simulink model "RC"  (R2020a)
settings: Solver=VariableStepAuto  StartTime=0.0  StopTime=30  FixedStep=0.2  RelTol=1e-3
values from neighbouring files (symbols this model uses):
  a = a+1    (= 1)    [rc_model.m]
  c = 1/10*10^-6    (= 1e-07)    [rc_model.m]
  r = 10    [rc_model.m]
settings Model: Creator=I3  LastModifiedBy=I3

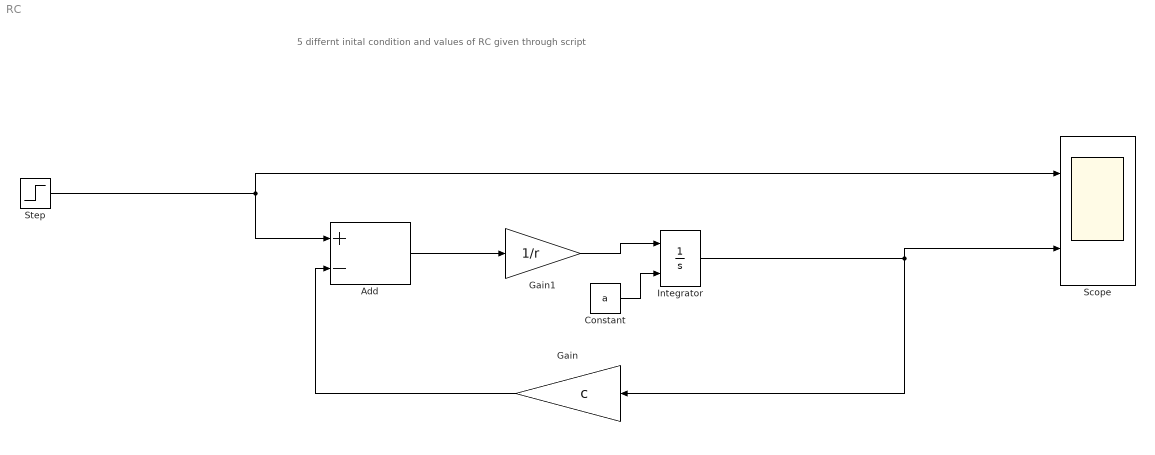
== system RC ==
  note: 5 differnt inital condition and values of RC given through script
  Add : Sum  Inputs=+-
  Constant : Constant  Value=a
  Gain : Gain  Gain=c
  Gain1 : Gain  Gain=1/r
  Integrator : Integrator  InitialConditionSource=external
  Scope : Scope  NumInputPorts=2
  Step : Step  SampleTime=0
  wires:
  Add/1 -> Gain1/1
  Integrator/1 -> Gain/1, Scope/2
  Gain/1 -> Add/2
  Gain1/1 -> Integrator/1
  Step/1 -> Scope/1, Add/1
  Constant/1 -> Integrator/2
